simulink subsystem "BackwardAccConverter"  (R2023a)
settings: Solver=VariableStepAuto  StartTime=0.0  StopTime=10.0  RelTol=1e-3
model mask{i_RackAndPinion=20, i_Gearbox=100}
  mask prompts: i_RackAndPinion "Rack and pinion transfer coeff (rad/mm)"; i_Gearbox "Gearbox reduction coeff"
settings Model: Creator=user  LastModifiedBy=user

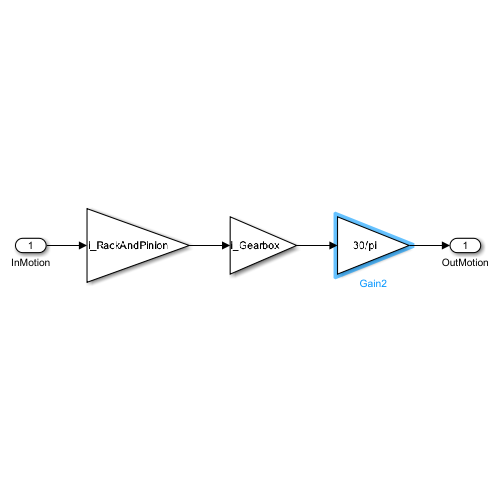
[thumbnail: Simulink's stored preview of the top-level diagram]
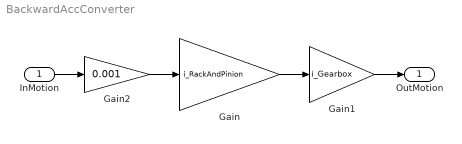
== system BackwardAccConverter ==
  InMotion : Inport
  Gain : Gain  Gain=i_RackAndPinion
  Gain1 : Gain  Gain=i_Gearbox
  Gain2 : Gain  Gain=0.001
  OutMotion : Outport
  wires:
  InMotion/1 -> Gain2/1
  Gain/1 -> Gain1/1
  Gain1/1 -> OutMotion/1
  Gain2/1 -> Gain/1
